simulink model "mreza"  (Simulink 5.0)
settings: Solver=ode23tb  SolverMode=SingleTasking  StartTime=0.0  StopTime=0.2  RelTol=1e-3
libraries: powerlib2 x13
settings Model: Creator=patrice  LastModifiedBy=yeti  ExtModeTrigMode=oneshot  ExtModeArmWhenConnect=off  LimitDataPoints=off  BlockReductionOpt=off  BooleanDataType=off  RTWTemplateMakefile=grt_unix.tmf

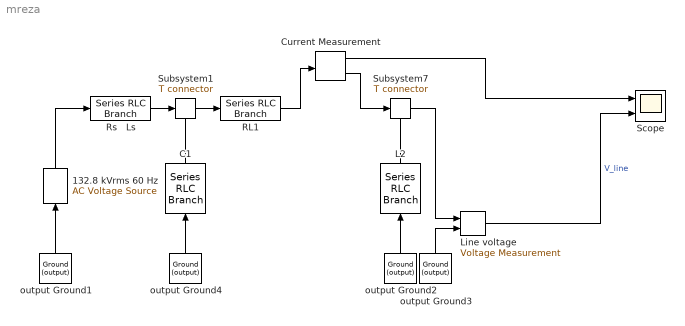
== system mreza ==
  132.8 kVrms 60 Hz : powerlib2/Electrical Sources/AC Voltage Source  Tag=PoWeRsYsTeMbLoCk  Orientation=up  A=230e3/sqrt(3)*sqrt(2)  P=90  F=60  stime=0  mesure=None  PSBOutputType=1
  C1 : powerlib2/Elements/Series RLC Branch  Tag=PoWeRsYsTeMbLoCk  Orientation=up  a=0  b=0  c=0.967e-06  mesure=None  PSBOutputType=1
  Current Measurement : powerlib2/Measurements/Current Measurement  Tag=PoWeRsYsTeMmEaSuReMeNt  PhasorSimulation=off  OutputType=Magnitude  PSBOutputType=01  PSBequivalent=0
  L2 : powerlib2/Elements/Series RLC Branch  Tag=PoWeRsYsTeMbLoCk  Orientation=up  a=0  b=1e-3  c=inf  mesure=None  PSBOutputType=1
  Line voltage : powerlib2/Measurements/Voltage Measurement  Tag=PoWeRsYsTeMmEaSuReMeNt  PhasorSimulation=off  OutputType=Magnitude  PSBOutputType=0  PSBequivalent=1
  RL1 : powerlib2/Elements/Series RLC Branch  Tag=PoWeRsYsTeMbLoCk  a=5.2  b=0  c=inf  mesure=None  PSBOutputType=1
  Rs   Ls : powerlib2/Elements/Series RLC Branch  Tag=PoWeRsYsTeMbLoCk  a=2.645  b=0  c=inf  mesure=None  PSBOutputType=1
  Scope : Scope  NumInputPorts=2
      settings: TimeRange=0.2  YMin=-40000~-10000  YMax=40000~10000  DataFormat=Array
  Subsystem1 : powerlib2/Connectors/T connector  Tag=PoWeRsYsTeMbLoCk  PSBOutputType=1
  Subsystem7 : powerlib2/Connectors/T connector  Tag=PoWeRsYsTeMbLoCk  PSBOutputType=1
  output Ground{1..4} (4 alike) : powerlib2/Connectors/Ground (output)  Tag=PoWeRsYsTeMbLoCk  Orientation=up  PSBOutputType=1
  wires:
  output Ground3/1 -> Line voltage/2
  Subsystem7/1 -> Line voltage/1
  output Ground2/1 -> L2/1
  L2/1 -> Subsystem7/Enable
  RL1/1 -> Current Measurement/1
  132.8 kVrms 60 Hz/1 -> Rs   Ls/1
  output Ground1/1 -> 132.8 kVrms 60 Hz/1
  Line voltage/1 -> Scope/2  "V_line"
  Rs   Ls/1 -> Subsystem1/1
  Subsystem1/1 -> RL1/1
  C1/1 -> Subsystem1/Enable
  output Ground4/1 -> C1/1
  Current Measurement/2 -> Subsystem7/1
  Current Measurement/1 -> Scope/1
